simulink model "p4"  (R2021b)
settings: Solver=VariableStepAuto  StartTime=0.0  StopTime=10.0  RelTol=1e-3
settings Model: Creator=brame  LastModifiedBy=brame

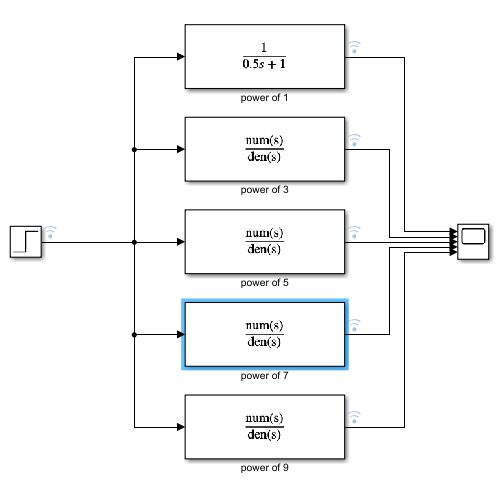
[thumbnail: Simulink's stored preview of the top-level diagram]
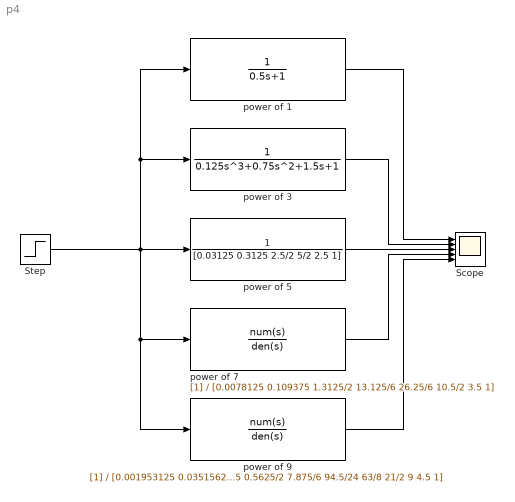
== system p4 ==
  Scope : Scope  NumInputPorts=5
  Step : Step  SampleTime=0
  power of 1 : TransferFcn  Denominator=[0.5 1]
  power of 3 : TransferFcn  Denominator=[0.125 0.75 1.5 1]
  power of 5 : TransferFcn  Denominator=[0.03125 0.3125 2.5/2 5/2 2.5 1]
  power of 7 : TransferFcn  Denominator=[0.0078125 0.109375 1.3125/2 13.125/6 26.25/6 10.5/2 3.5 1]
  power of 9 : TransferFcn  Denominator=[0.001953125 0.03515625 0.5625/2 7.875/6 94.5/24 63/8 21/2 9 4.5 1]
  wires:
  Step/1 -> power of 1/1, power of 3/1, power of 5/1, power of 7/1, power of 9/1
  power of 1/1 -> Scope/1
  power of 3/1 -> Scope/2
  power of 5/1 -> Scope/3
  power of 7/1 -> Scope/4
  power of 9/1 -> Scope/5
